simulink model "chap16_9sim"  (Simulink 8.3)
settings: Solver=ode45  StartTime=0.0  StopTime=2  FixedStep=0.001  RelTol=1e-3
settings Model: Creator=hp  LastModifiedBy=Administrator
settings DataIOCC: SignalLoggingName=sigsOut
settings OptimizationCC: ExpressionDepthLimit=2147483647  InitFltsAndDblsToZero=on
settings DebuggingCC: SaveWithParameterizedLinksMsg=none  SignalResolutionControl=TryResolveAllWithWarning  SolverPrmCheckMsg=none  MultiTaskDSMMsg=warning  MultiTaskCondExecSysMsg=none  FcnCallInpInsideContextMsg=UseLocalSettings
settings HardwareCC: TargetUnknown=on
settings RTWCC: IncludeERTFirstTime=on
settings GRTTargetCC: TargetFcnLib=ansi_tfl_tmw.mat

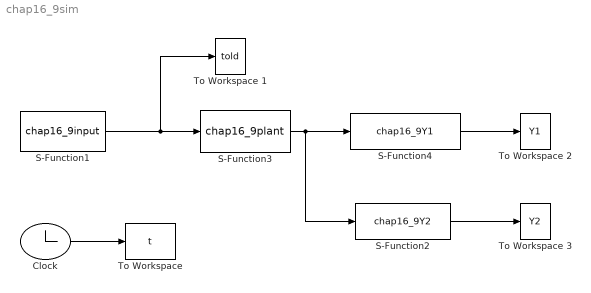
== system chap16_9sim ==
  Clock : Clock
  S-Function1 : S-Function  FunctionName=chap16_9input  EnableBusSupport=off
  S-Function2 : S-Function  FunctionName=chap16_9Y2  EnableBusSupport=off
  S-Function3 : S-Function  FunctionName=chap16_9plant  EnableBusSupport=off
  S-Function4 : S-Function  FunctionName=chap16_9Y1  EnableBusSupport=off
  To Workspace : ToWorkspace  VariableName=t  SampleTime=-1
  To Workspace 1 : ToWorkspace  VariableName=told  SampleTime=-1
  To Workspace 2 : ToWorkspace  VariableName=Y1  SampleTime=-1
  To Workspace 3 : ToWorkspace  VariableName=Y2  SampleTime=-1
  wires:
  Clock/1 -> To Workspace/1
  S-Function3/1 -> S-Function4/1, S-Function2/1
  S-Function4/1 -> To Workspace 2/1
  S-Function2/1 -> To Workspace 3/1
  S-Function1/1 -> S-Function3/1, To Workspace 1/1
